simulink model "raddi_est_2016b"  (R2016b)
settings: Solver=ode45  StartTime=0.0  StopTime=inf  RelTol=1e-3  EnableMultiTasking=on
settings Model: Creator=igeorgie  LastModifiedBy=igeorgie
settings DataIOCC: LimitDataPoints=on  SaveFormat=Array
settings OptimizationCC: LifeSpan=inf
settings DebuggingCC: UnderspecifiedInitializationDetection=Classic  MergeDetectMultiDrivingBlocksExec=none  SolverPrmCheckMsg=warning  SFUnexpectedBacktrackingDiag=warning  SFNoUnconditionalDefaultTransitionDiag=warning  SFExecutionAtInitializationDiag=none
settings HardwareCC: ProdBitPerPointer=32  ProdBitPerSizeT=32  ProdBitPerPtrDiffT=32  ProdLargestAtomicFloat=None  ProdIntDivRoundTo=Undefined  ProdEndianess=Unspecified  ProdWordSize=32  ProdHWDeviceType=32-bit Generic
settings ModelReferenceCC: PropagateSignalLabelsOutOfModel=off
settings GRTTargetCC: TargetLangStandard=C89/C90 (ANSI)  GeneratePreprocessorConditionals=Disable all
settings ConfigComp: CovMetricSettings=dw  CovHtmlReporting=on  CovSaveCumulativeToWorkspaceVar=on  CovSaveSingleToWorkspaceVar=on  CovExternalEMLEnable=off

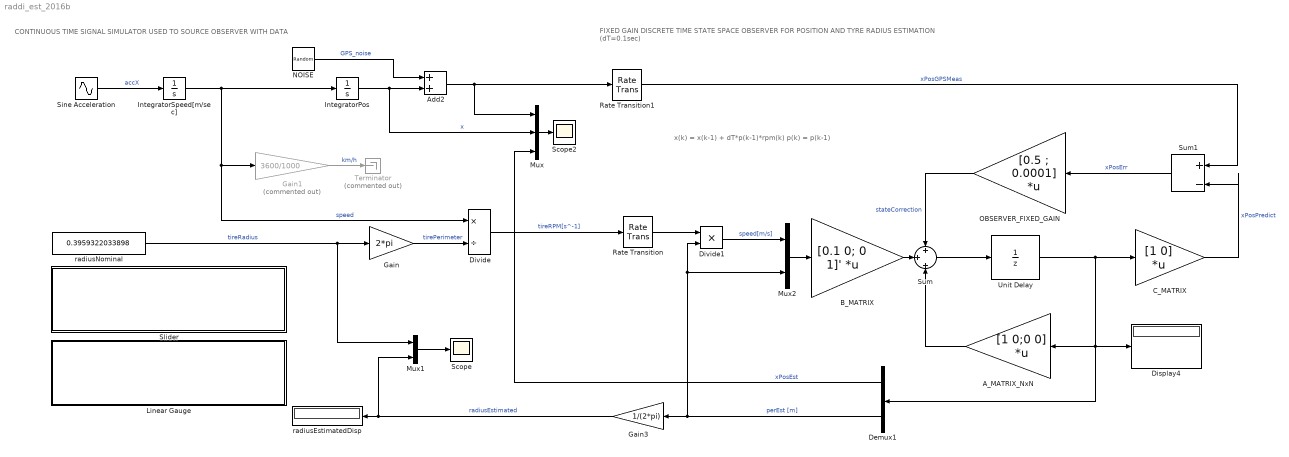
== system raddi_est_2016b ==
  note: x(k) = x(k-1) + dT*p(k-1)*rpm(k)
      | p(k) = p(k-1)
  note: CONTINUOUS TIME SIGNAL SIMULATOR USED TO SOURCE OBSERVER WITH DATA
  note: FIXED GAIN DISCRETE TIME STATE SPACE OBSERVER FOR POSITION AND TYRE RADIUS ESTIMATION (dT=0.1sec)
  A_MATRIX_NxN : Gain  Gain=[1 0;0 0]  Multiplication=Matrix(K*u)
  Add2 : Sum
  B_MATRIX : Gain  Gain=[0.1 0; 0 1]'  Multiplication=Matrix(K*u)
  C_MATRIX : Gain  Gain=[1 0]  Multiplication=Matrix(K*u)
  Demux1 : Demux  Outputs=2
  Display4 : Display
  Divide : Product  Inputs=*/
  Divide1 : Product  Inputs=**
  Gain : Gain  Gain=2*pi
  Gain1 : Gain  Commented=on  Gain=3600/1000
  Gain3 : Gain  Gain=1/(2*pi)
  IntegratorPos : Integrator
  IntegratorSpeed[m/sec] : Integrator
  Linear Gauge : Subsystem  DialogController=hmiCreateDDGDialog  IsWebBlock=on  mask(MWDashboardBlock){webBlockId=3646f1cb-7a87-4cc7-ac23-8b65aa10fd2d, webBlockType=lineargauge, ShowInLibBrowser=on, ShowInitialText=on, HMISrcModelName=raddi_est_2016b}
      mask prompts: webBlockId "WebBlock Id"; webBlockType "WebBlock Type"; HMISrcModelName "Source Model"
      mask help: SimulinkHMI:dialogs:LinearGaugeDialogDesc
      mask Help: helpview([docroot '/mapfiles/simulink.map'], 'hmi_linear_gauge')
      mask Display:
      | if strcmp(get_param(bdroot(gcb),'BlockDiagramType'), 'library')
      |     image([(matlabroot) '/toolbox/simulink/hmi/icons/LinearGauge.png']);
      | end
  Mux : Mux  Inputs=3
  Mux1 : Mux  Inputs=2
  Mux2 : Mux  Inputs=2
  NOISE : RandomNumber  Variance=2000  SampleTime=0.1
  OBSERVER_FIXED_GAIN : Gain  Gain=[0.5 ; 0.0001]  Multiplication=Matrix(K*u)
  Rate Transition : RateTransition  OutPortSampleTime=0.1
  Rate Transition1 : RateTransition  OutPortSampleTime=0.1
  Scope : Scope
  Scope2 : Scope
  Sine Acceleration : Sin  Amplitude=0.03  Frequency=2*pi*(1/3600)
  Slider : Subsystem  DialogController=hmiCreateDDGDialog  IsWebBlock=on  mask(MWDashboardBlock){webBlockId=42f85781-b5a0-4525-a9ad-210628367d4a, webBlockType=slider, ShowInLibBrowser=on, ShowInitialText=on, HMISrcModelName=raddi_est_2016b}
      mask prompts: webBlockId "WebBlock Id"; webBlockType "WebBlock Type"; HMISrcModelName "Source Model"
      mask help: SimulinkHMI:dialogs:SliderDialogDesc
      mask Help: helpview([docroot '/mapfiles/simulink.map'], 'hmi_slider')
      mask Display:
      | if strcmp(get_param(bdroot(gcb),'BlockDiagramType'), 'library')
      |     image([(matlabroot) '/toolbox/simulink/hmi/icons/Slider.png']);
      | end
  Sum : Sum  Inputs=+|+|+
  Sum1 : Sum  Inputs=+-|
  Terminator : Terminator  Commented=on
  Unit Delay : UnitDelay  InitialCondition=[1000 2]  SampleTime=-1
  radiusEstimatedDisp : Display
  radiusNominal : Constant  Value=0.3959322033898
  wires:
  Sine Acceleration/1 -> IntegratorSpeed[m/sec]/1  "accX"
  IntegratorPos/1 -> Mux/2, Add2/2  "x"
  IntegratorSpeed[m/sec]/1 -> IntegratorPos/1, Divide/1, Gain1/1  "speed"
  Gain/1 -> Divide/2  "tirePerimeter"
  radiusNominal/1 -> Gain/1, Mux1/1  "tireRadius"
  Divide/1 -> Rate Transition/1  "tireRPM[s^-1]"
  Rate Transition/1 -> Divide1/1
  A_MATRIX_NxN/1 -> Sum/3
  Sum/1 -> Unit Delay/1
  Unit Delay/1 -> Demux1/1, Display4/1, A_MATRIX_NxN/1, C_MATRIX/1
  C_MATRIX/1 -> Sum1/2  "xPosPredict"
  Sum1/1 -> OBSERVER_FIXED_GAIN/1  "xPosErr"
  OBSERVER_FIXED_GAIN/1 -> Sum/1  "stateCorrection"
  Mux/1 -> Scope2/1
  Demux1/1 -> Mux/3  "xPosEst"
  Demux1/2 -> Mux2/2, Divide1/2, Gain3/1  "perEst [m]"
  Rate Transition1/1 -> Sum1/1  "xPosGPSMeas"
  B_MATRIX/1 -> Sum/2
  Divide1/1 -> Mux2/1  "speed[m/s]"
  Mux2/1 -> B_MATRIX/1
  Add2/1 -> Mux/1, Rate Transition1/1
  NOISE/1 -> Add2/1  "GPS_noise"
  Gain3/1 -> Mux1/2, radiusEstimatedDisp/1  "radiusEstimated"
  Mux1/1 -> Scope/1
  Gain1/1 -> Terminator/1  "km/h"

== system raddi_est_2016b/Linear Gauge ==

== system raddi_est_2016b/Slider ==
